simulink model "sim_5_dc_motor"  (R2022b)
settings: Solver=VariableStepAuto  StartTime=0.0  StopTime=10.0  RelTol=1e-3
values from neighbouring files (symbols this model uses):
  b = 0.2    [dc_params.mat]    (also in sim_5_dc_param.m)
  J = 0.02    [dc_params.mat]    (also in sim_5_dc_param.m)
  K_e = 0.1    [dc_params.mat]    (also in sim_5_dc_param.m)
  K_t = 0.1    [dc_params.mat]    (also in sim_5_dc_param.m)
  L = 0.5    [dc_params.mat]    (also in sim_5_dc_param.m)
  R = 2    [dc_params.mat]    (also in sim_5_dc_param.m)
settings Model: Creator=user  LastModifiedBy=user

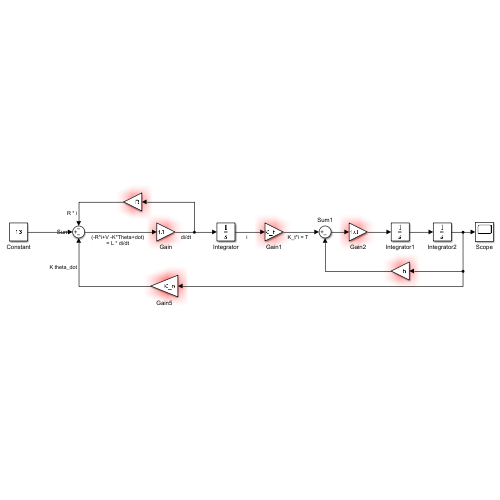
[thumbnail: Simulink's stored preview of the top-level diagram]
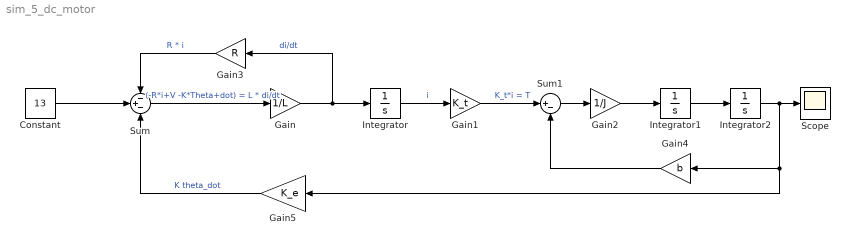
== system sim_5_dc_motor ==
  Constant : Constant  Value=13
  Gain : Gain  Gain=1/L
  Gain1 : Gain  Gain=K_t
  Gain2 : Gain  Gain=1/J
  Gain3 : Gain  Gain=R
  Gain4 : Gain  Gain=b
  Gain5 : Gain  Gain=K_e
  Integrator : Integrator
  Integrator1 : Integrator
  Integrator2 : Integrator
  Scope : Scope
  Sum : Sum  Inputs=-+-
  Sum1 : Sum  Inputs=|+-
  wires:
  Constant/1 -> Sum/2
  Gain3/1 -> Sum/1  "R * i"
  Gain5/1 -> Sum/3  "K theta_dot"
  Sum/1 -> Gain/1  "(-R*i+V -K*Theta+dot) = L * di/dt"
  Gain/1 -> Gain3/1, Integrator/1  "di/dt"
  Integrator/1 -> Gain1/1  "i"
  Gain1/1 -> Sum1/1  "K_t*i = T"
  Sum1/1 -> Gain2/1
  Gain2/1 -> Integrator1/1
  Integrator1/1 -> Integrator2/1
  Integrator2/1 -> Gain5/1, Gain4/1, Scope/1
  Gain4/1 -> Sum1/2
